simulink model "Main"  (Simulink 6.6)
settings: Solver=FixedStepDiscrete  StartTime=0.0  StopTime=Inf  FixedStep=0.001  RelTol=1e-3
undefined symbols (not defined in the file): ecan1_init, ecan1_receive_matlab, ecan1_transmit_matlab, u1, y1
libraries: simulink x83, dsPICdrivers x6
(part 1 of 2)
CloseFcn:
  | rtwprivate ssgencode ModelCloseRequest Main
settings Model: Creator=bwmairs  LastModifiedBy=bwmairs  ProdHWDeviceType=16-bit Generic
settings OptimizationCC: InlineParams=on  OptimizeModelRefInitCode=on  LifeSpan=1
settings HardwareCC: ProdBitPerInt=16  ProdEndianess=LittleEndian  ProdWordSize=16  ProdHWDeviceType=16-bit Generic  TargetHWDeviceType=32-bit Generic
settings RTWCC: SystemTargetFile=dspic.tlc  TemplateMakefile=dspic_pic30_gcc.tmf  PostCodeGenCommand=dsPIC_Compile()  Description=Embedded Target for Microchip dsPIC (real-time)  ProcessScript=dspic_make_rtw_hook
settings RTWCC: CustomSource=|
  | ../../circBuffer.c
  | ../../ecanFunctions.c
settings CodeAppCC: IgnoreCustomStorageClasses=off
settings STFCustomTargetCC: TargetFcnLib=ansi_tfl_tmw.mat  GenFloatMathFcnCalls=ANSI_C  ModelReferenceCompliant=off  IncludeMdlTerminateFcn=off  CombineOutputUpdateFcns=on  SuppressErrorStatus=on  ERTCustomFileBanners=on  SupportContinuousTime=off  SupportNonInlinedSFcns=off  SystemTargetFile=dspic.tlc
settings ERTTargetCC: TargetFcnLib=ansi_tfl_tmw.mat  GenFloatMathFcnCalls=ANSI_C  ModelReferenceCompliant=off  IncludeMdlTerminateFcn=off  SuppressErrorStatus=on  ModelStepFunctionPrototypeControlCompliant=off  ExtModeMexFile=noextcomm  InlinedParameterPlacement=NonHierarchical  ERTSrcFileBannerTemplate=dsPIC_code_template.cgt  ERTHdrFileBannerTemplate=dsPIC_code_template.cgt  ERTDataSrcFileTemplate=dsPIC_code_template.cgt  ERTDataHdrFileTemplate=dsPIC_code_template.cgt  ERTCustomFileTemplate=dsPIC_main.tlc
settings CustomProperty: DataType=string  Value=C:\PROGRA~1\MATLAB\R2007a\rtw\bin\win32\gmake

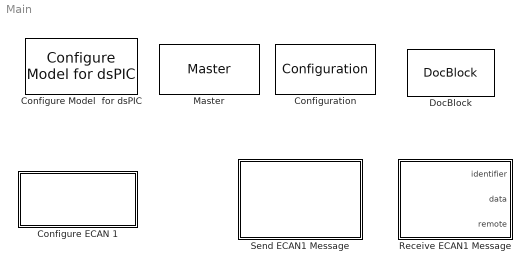
== system Main ==
  Configuration : dsPICdrivers/Configuration  SystemSampleTime=-1  double64=off
  Configure ECAN 1 : Subsystem  mask(Initialize ECAN 1){frame_setting=off, mode=Normal, dma_rx_chan=2, dma_tx_chan=0, baud=2500, cpu_freq=40000, ps1=8, pd=5, ps2=6, sjw=3, tq=20, triple_sample=on, dma_buf_size=4 buffers, rx_bufs=[0], tx_bufs=[1], buf_0_tx_pri=Highest, buf_0_rte=No, buf_1_tx_pri=Highest, buf_1_rte=No, buf_2_tx_pri=Lowest, buf_2_rte=No, buf_3_tx_pri=Lowest, buf_3_rte=No, buf_4_tx_pri=Lowest, buf_4_rte=No, buf_5_tx_pri=Lowest, buf_5_rte=No, buf_6_tx_pri=Lowest, buf_6_rte=No, buf_7_tx_pri=Lowest, buf_7_rte=No, mask_0=0, mask_0_rm=0, mask_1=0, mask_1_rm=0, mask_2=0, mask_2_rm=0, filters=[0 1 2], filter_0=hex2dec('400'), filter_0_mask=1, filter_0_exide=off, filter_0_buf=1, filter_1=hex2dec('401'), filter_1_mask=1, filter_1_exide=off, filter_1_buf=1, filter_2=hex2dec('402'), filter_2_mask=1, filter_2_exide=off, filter_2_buf=1, filter_3=0, filter_3_mask=0, filter_3_exide=off, filter_3_buf=0, filter_4=0, filter_4_mask=0, filter_4_exide=0, filter_4_buf=0, filter_5=0, filter_5_mask=0, filter_5_exide=off, filter_5_buf=0, filter_6=0, filter_6_mask=0, filter_6_exide=off, filter_6_buf=0, filter_7=0, filter_7_mask=0, filter_7_exide=off, filter_7_buf=0, filter_8=0, filter_8_mask=0, filter_8_exide=off, filter_8_buf=0, filter_9=0, filter_9_mask=0, filter_9_exide=off, filter_9_buf=0, filter_10=0, filter_10_mask=0, filter_10_exide=off, filter_10_buf=0, filter_11=0, filter_11_mask=0, filter_11_exide=off, filter_11_buf=0, filter_12=0, filter_12_mask=0, filter_12_exide=off, filter_12_buf=0, filter_13=0, filter_13_mask=0, filter_13_exide=off, filter_13_buf=0, filter_14=0, filter_14_mask=0, filter_14_exide=off, filter_14_buf=0, filter_15=0, filter_15_mask=0, filter_15_exide=off, filter_15_buf=0}
      mask prompts: frame_setting "Extended Frames (Standard if unchecked)"; dma_rx_chan "DMA Reception Channel"; dma_tx_chan "DMA Transmission Channel"; baud "Baud Rate (hundreds of bps)"; cpu_freq "CPU Frequency (in kHz)"; ps1 "Phase Segment 1"; pd "Propagation Delay"; ps2 "Phase Segment 2"; sjw "Sync Jump Width"; tq "Time Quanta"; triple_sample "Triple-sample"; dma_buf_size "DMA Buffer Size"; rx_bufs "Reception Buffers"; tx_bufs "Transmission Buffers"; buf_0_tx_pri "Buffer 0 Transmission Priority"; buf_0_rte "Buffer 0 Remote Transmit Enable"; buf_1_tx_pri "Buffer 1 Transmission Priority"; buf_1_rte "Buffer 1 Remote Transmit Enable"; buf_2_tx_pri "Buffer 2 Transmission Priority"; buf_2_rte "Buffer 2 Remote Transmit Enable"; buf_3_tx_pri "Buffer 3 Transmission Priority"; buf_3_rte "Buffer 3 Remote Transmit Enable"; buf_4_tx_pri "Buffer 4 Transmission Priority"; buf_4_rte "Buffer 4 Remote Transmit Enable"; buf_5_tx_pri "Buffer 5 Transmission Priority"; buf_5_rte "Buffer 5 Remote Transmit Enable"; buf_6_tx_pri "Buffer 6 Transmission Priority"; buf_6_rte "Buffer 6 Remote Transmit Enable"; buf_7_tx_pri "Buffer 7 Transmission Priority"; buf_7_rte "Buffer 7 Remote Transmit Enable"; mask_0 "Mask 0"; mask_0_rm "Mask 0 Receive Mode"; mask_1 "Mask 1"; mask_1_rm "Mask 1 Receive Mode"; mask_2 "Mask 2"; mask_2_rm "Mask 2 Receive Mode"; filter_0 "Filter 0"; filter_0_mask "Filter 0 Mask"; filter_0_exide "Filter 0 Extended Enable"; filter_0_buf "Filter 0 Buffer"; filter_1 "Filter 1"; filter_1_mask "Filter 1 Mask"; filter_1_exide "Filter 1 Extended Enable"; filter_1_buf "Filter 1 Buffer"; filter_2 "Filter 2"; filter_2_mask "Filter 2 Mask"; filter_2_exide "Filter 2 Extended Enable"; filter_2_buf "Filter 2 Buffer"; filter_3 "Filter 3"; filter_3_mask "Filter 3 Mask"; filter_3_exide "Filter 3 Extended Enable"; filter_3_buf "Filter 3 Buffer"; filter_4 "Filter 4"; filter_4_mask "Filter 4 Mask"; filter_4_exide "Filter 4 Extended Enable"; filter_4_buf "Filter 4 Buffer"; filter_5 "Filter 5"; filter_5_mask "Filter 5 Mask"; filter_5_exide "Filter 5 Extended Enable"; filter_5_buf "Filter 5 Buffer"; filter_6 "Filter 6"; filter_6_mask "Filter 6 Mask"; filter_6_exide "Filter 6 Extended Enable"; filter_6_buf "Filter 6 Buffer"; filter_7 "Filter 7"; filter_7_mask "Filter 7 Mask"; filter_7_exide "Filter 7 Extended Enable"; filter_7_buf "Filter 7 Buffer"; filter_8 "Filter 8"; filter_8_mask "Filter 8 Mask"; filter_8_exide "Filter 8 Extended Enable"; filter_8_buf "Filter 8 Buffer"; filter_9 "Filter 9"; filter_9_mask "Filter 9 Mask"; filter_9_exide "Filter 9 Extended Enable"; filter_9_buf "Filter 9 Buffer"; filter_10 "Filter 10"; filter_10_mask "Filter 10 Mask"; filter_10_exide "Filter 10 Extended Enable"; filter_10_buf "Filter 10 Buffer"; filter_11 "Filter 11"; filter_11_mask "Filter 11 Mask"; filter_11_exide "Filter 11 Extended Enable"; filter_11_buf "Filter 11 Buffer"; filter_12 "Filter 12"; filter_12_mask "Filter 12 Mask"; filter_12_exide "Filter 12 Extended Enable"; filter_12_buf "Filter 12 Buffer"; filter_13 "Filter 13"; filter_13_mask "Filter 13 Mask"; filter_13_exide "Filter 13 Extended Enable"; filter_13_buf "Filter 13 Buffer"; filter_14 "Filter 14"; filter_14_mask "Filter 14 Mask"; filter_14_exide "Filter 14 Extended Enable"; filter_14_buf "Filter 14 Buffer"; filter_15 "Filter 15"; filter_15_mask "Filter 15 Mask"; filter_15_exide "Filter 15 Extended Enable"; filter_15_buf "Filter 15 Buffer"
      mask help: Initializes the ECAN 1 module on the dsPIC33f. Allows for configuration of almost all ECAN options to produce a usable system.
      mask StyleString: checkbox,popup(Normal|Disabled|Loopback|Listen only|Configuration|UNDEFINED|UNDEFINED|Listen all),edit,edit,edit,edit,edit,edit,edit,popup(0|1|2|3),edit,checkbox,popup(4 buffers|6 buffers|8 buffers|12 buffers|16 buffers|24 buffers|32 buffers),edit,edit,popup(Lowest|Low|High|Highest),popup(No|Yes),popup(Lowest|Low|High|Highest),popup(No|Yes),popup(Lowest|Low|High|Highest),popup(No|Yes),popup(Lowest|Low|High|Highest),popup(No|Yes),popup(Lowest|Low|High|Highest),popup(No|Yes),popup(Lowest|Low|High|Highest),popup(No|Yes),popup(Lowest|Low|High|Highest),popup(No|Yes),popup(Lowest|Low|High|Highest),popup(No|Yes),edit,popup(0|1),edit,popup(0|1),edit,popup(0|1),edit,edit,popup(--|0|1|2),checkbox,popup(0|1|2|3|4|5|6|7|8|9|10|11|12|13|14|FIFO),edit,popup(0|1|2|--),checkbox,popup(0|1|2|3|4|5|6|7|8|9|10|11|12|13|14|FIFO),edit,popup(0|1|2|--),checkbox,popup(0|1|2|3|4|5|6|7|8|9|10|11|12|13|14|FIFO),edit,popup(0|1|2|--),checkbox,popup(0|1|2|3|4|5|6|7|8|9|10|11|12|13|14|FIFO),edit,popup(0|1|2|--),edit,popup(0|1|2|3|4|5|6|7|8|9|10|11|12|13|14|FIFO),edit,popup(0|1|2|--),checkbox,popup(0|1|2|3|4|5|6|7|8|9|10|11|12|13|14|FIFO),edit,popup(0|1|2|--),checkbox,popup(0|1|2|3|4|5|6|7|8|9|10|11|12|13|14|FIFO),edit,popup(0|1|2|--),checkbox,popup(0|1|2|3|4|5|6|7|8|9|10|11|12|13|14|FIFO),edit,popup(0|1|2|--),checkbox,popup(0|1|2|3|4|5|6|7|8|9|10|11|12|13|14|FIFO),edit,popup(0|1|2|--),checkbox,popup(0|1|2|3|4|5|6|7|8|9|10|11|12|13|14|FIFO),edit,popup(0|1|2|--),checkbox,popup(0|1|2|3|4|5|6|7|8|9|10|11|12|13|14|FIFO),edit,popup(0|1|2|--),checkbox,popup(0|1|2|3|4|5|6|7|8|9|10|11|12|13|14|FIFO),edit,popup(0|1|2|--),checkbox,popup(0|1|2|3|4|5|6|7|8|9|10|11|12|13|14|FIFO),edit,popup(0|1|2|--),checkbox,popup(0|1|2|3|4|5|6|7|8|9|10|11|12|13|14|FIFO),edit,popup(0|1|2|--),checkbox,popup(0|1|2|3|4|5|6|7|8|9|10|11|12|13|14|FIFO),edit,popup(0|1|2|--),checkbox,popup(0|1|2|3|4|5|6|7|8|9|10|11|12|13|14|FIFO)
      mask CallbackString:
      | ||||||tq = 1 + str2num(get_param(gcb, 'ps1')) + str2num(get_param(gcb, 'pd')) + str2num(get_param(gcb, 'ps2'));
      | set_param(gcb, 'tq', int2str(tq));|tq = 1 + str2num(get_param(gcb, 'ps1')) + str2num(get_param(gcb, 'pd')) + str2num(get_param(gcb, 'ps2'));
      | set_param(gcb, 'tq', int2str(tq));|tq = 1 + str2num(get_param(gcb, 'ps1')) + str2num(get_param(gcb, 'pd')) + str2num(get_param(gcb, 'ps2'));
      | set_param(gcb, 'tq', int2str(tq));||||||filters = eval(get_param(gcb,'tx_bufs'));
      | mVisibilities = get_param(gcb,'MaskVisibilities');
      | mNames = get_param(gcb,'MaskNames');
      | for i = 1:size(mNames);
      | 	n = mNames{i};
      |     if size(n,2) > 4 && strcmp(n(1:4), 'buf_') == 1
      |         filterNumber = sscanf(n, 'buf_%d');
      |         if isempty(find(filters == filterNumber, 1)) == 0
      |              mVisibilities{i} = 'on';
      |         else
      |              mVisibilities{i} = 'off';
      |         end
      |     end
      | end
      | set_param(gcb, 'MaskVisibilities', mVisibilities);|||||||||||||||||||||||filters = eval(get_param(gcb,'filters'));
      | mVisibilities = get_param(gcb,'MaskVisibilities');
      | mNames = get_param(gcb,'MaskNames');
      | for i = 1:size(mNames);
      | 	n = mNames{i};
      |     if size(n,2) > 7 && strcmp(n(1:7), 'filter_') == 1
      |         filterNumber = sscanf(n, 'filter_%d');
      |         if isempty(find(filters == filterNumber, 1)) == 0
      |              mVisibilities{i} = 'on';
      |         else
      |              mVisibilities{i} = 'off';
      |         end
      |     end
      | end
      | set_param(gcb, 'MaskVisibilities', mVisibilities);||||||||||||||||||||||||||||||||||||||||||||||||||||||||||||||||
      mask Display: text(0.5,0.5,'Configure ECAN1','horizontalAlignment','center','verticalAlignment','middle');
  Configure Model  for dsPIC : dsPICdrivers/Simulink Configuration/Configure Model  for dsPIC
  DocBlock : simulink/Model-Wide Utilities/DocBlock  SystemSampleTime=-1  DocumentType=Text
      content=|
      | This model recreates the Crosswire application note from Microchip.
      | The Debugging directory includes an MPLAB project that can compile and load
      | the MATLAB-generated code in order to facilitate debugging.
  Master : dsPICdrivers/Master  Tag=dsPIC_MASTER  Priority=1  TimeStepType=Timer1  picType=33fJ256GP710  fcy=40000000  Quartz_33f=8e6  PLLActive_33f=on  fcyDesired_33f=40000000  tmr1="[1  39999  0]"  tmr1Info="Time Step : 0.001  ;   Error : 0%  PR1=39999"  tmr2345="[0  0  0  0  0  0  0  0]"  tmr2345cfg=[-1 -1 -1 -1 -1 -1 -1 -1]  IOautoConf=on  typePort="[ 0  0  0  0  0  0  0  0  0  0  0  0  0  0  0  0  0  0  0  0  0  0  0  0  0  0  0  0  0  0  0  0  0  0  0  0  0  0  0  0  0  0  0  0  0  0  0  0  0  0  0  0  0  0  0  0  0  0  0  0  0  0  0  0  0  0  0  0  0  0  0  0  0  0  0  0  0  0  0  0  0  0  0  0  0  0  0  0  0  0  0  0  0  0  0  0  0  0  0  0  0  0  0  0  0  0  0  0  0  0  0  0 ]"  TRIS="[ 65535  65535  65535  65535  65535  65535  65535 ]"  ADPCFG=0  MasterBusyPort=None  MasterOverloadPort=None  FOSC=Quartz (XT - HS)  ClockSwitchMonitor=Both disabled  TempProtection_33f=TEMP_ON  FPBOR=<empty>  PWRT=disable  MCLR=<empty>  PowerSave=off  OverrideFcy=off  NewFcy=1e6  PR2345="[65535  65535  65535  65535  65535  65535  65535  65535]"
  Receive ECAN1 Message : Subsystem
  Send ECAN1 Message : Subsystem  mask(Send ECAN Message){buffer=1, identifier=hex2dec('401'), identifier_from_input=off, ide=off, remote=off, length=4, data=[hex2dec('11') hex2dec('12') hex2dec('13') hex2dec('14')], data_from_input=off, c_func_sample_time=1, trigger_on_input=off}
      mask prompts: identifier_from_input "Indentifier from input"; length "Data Length (bytes)"; data_from_input "Data from input"; c_func_sample_time "Sample time"; trigger_on_input "Trigger on input"
      mask help: This block allows for the transmission of a message over the ECAN module.
      mask CallbackString:
      | ||mEnables = get_param(gcb,'MaskEnables');
      | enabled = get_param(gcb, 'identifier_from_input');
      | if strcmp(enabled,'on');
      |     replace_block([gcb '/identifier'],'Constant','Inport','noprompt');
      |     mEnables{2} = 'off';
      |     set_param([gcb '/identifier'],'Port','1');
      | else
      |     replace_block([gcb '/identifier'],'Inport','Constant','noprompt');
      |     mEnables{2} = 'on';
      |     set_param([gcb '/identifier'],'Value','identifier');
      | end
      | set_param(gcb, 'MaskEnables', mEnables);
      | ||||data = eval(get_param(gcb, 'data'));
      | y = size(data,1);
      | x = size(data,2);
      | if y > 1 && x > 1
      |     error('Data must be a 1-dimensional vector')
      | else
      |     if or(x > 8, y > 8)
      |     error('Data cannot be larger than 8-bytes');
      |     end
      | end|mEnables = get_param(gcb,'MaskEnables');
      | enabled = get_param(gcb, 'data_from_input');
      | if strcmp(enabled,'on');
      |     mEnables{7} = 'off';
      |     replace_block([gcb '/data'],'Constant','Inport','noprompt');
      |     if strcmp(get_param([gcb '/identifier'],'BlockType'), 'Inport');
      |         set_param([gcb '/data'],'Port','2');
      |     else
      |         set_param([gcb '/data'],'Port','1');
      |     end
      | else
      |     mEnables{7} = 'on';
      |     replace_block([gcb '/data'],'Inport','Constant','noprompt');
      |     set_param([gcb '/data'],'Value','data');
      | end
      | set_param(gcb, 'MaskEnables', mEnables);||mEnables = get_param(gcb,'MaskEnables');
      | enabled = get_param(gcb, 'trigger_on_input');
      | if strcmp(enabled,'on');
      |     mEnables{9} = 'off';
      |     set_param([gcb '/C-function Call/ECAN1 Transmit'],'SampleTime','-1');
      |     replace_block([gcb '/trigger'],'Constant','Inport','noprompt');
      | else
      |     mEnables{9} = 'on';
      |     set_param([gcb '/C-function Call/ECAN1 Transmit'],'SampleTime','c_func_sample_time');
      |     replace_block([gcb '/trigger'],'Inport','Constant','noprompt');
      |     set_param([gcb '/trigger'],'Value','1');
      | end
      | set_param(gcb, 'MaskEnables', mEnables);
      mask Display: disp('ECAN1 TX');

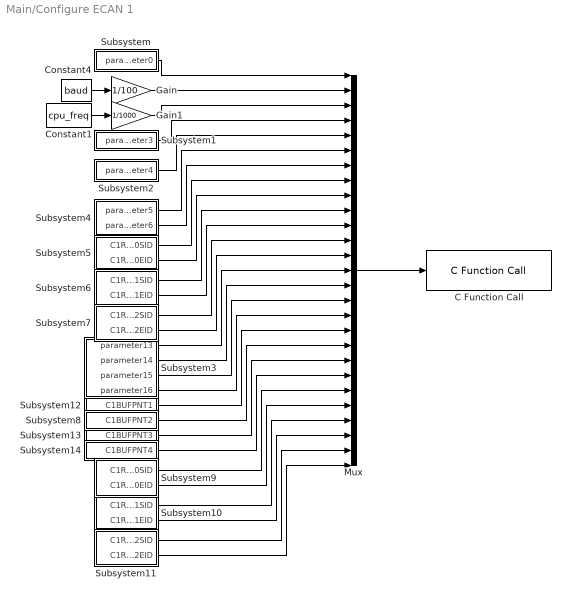
== system Main/Configure ECAN 1 ==
  C Function Call : dsPICdrivers/OTHERS/C Function Call  Tag=dsPIC_dsPIC_CFunctionCall  fctName='ecan1_init'  INPUT_SIZE=27  INPUT1=uint16  INPUT2=--  INPUT3=--  OUTPUT_SIZE=1  OUTPUT1=--  SampleTime=Inf  InputType=[ 4 ]  OutputType=[ ]  FctDeclaration=extern void ecan1_init(uint16_T* u1);  FctCall=ecan1_init(*%u1);  OrderingInOutPopup=None
  Constant1 : Constant  Value=cpu_freq  OutDataTypeMode=uint32
  Constant4 : Constant  Value=baud  OutDataTypeMode=uint32
  Gain : Gain  Gain=1/100  ParameterDataType=uint(16)  OutDataType=uint(16)
  Gain1 : Gain  Gain=1/1000  ParameterDataType=uint(16)
  Mux : Mux  Inputs=27
  Subsystem : Subsystem
  Subsystem1 : Subsystem
  Subsystem10 : Subsystem
  Subsystem11 : Subsystem
  Subsystem12 : Subsystem
  Subsystem13 : Subsystem
  Subsystem14 : Subsystem
  Subsystem2 : Subsystem
  Subsystem3 : Subsystem
  Subsystem4 : Subsystem
  Subsystem5 : Subsystem
  Subsystem6 : Subsystem
  Subsystem7 : Subsystem
  Subsystem8 : Subsystem
  Subsystem9 : Subsystem
  wires:
  Constant4/1 -> Gain/1
  Subsystem/1(parameter0) -> Mux/1
  Gain/1 -> Mux/2
  Subsystem1/1(parameter3) -> Mux/4
  Subsystem2/1(parameter4) -> Mux/5
  Subsystem4/2(parameter6) -> Mux/7
  Subsystem4/1(parameter5) -> Mux/6
  Subsystem5/1(C1RXM0SID) -> Mux/8
  Subsystem5/2(C1RXM0EID) -> Mux/9
  Subsystem6/1(C1RXM1SID) -> Mux/10
  Subsystem6/2(C1RXM1EID) -> Mux/11
  Subsystem7/1(C1RXM2SID) -> Mux/12
  Subsystem7/2(C1RXM2EID) -> Mux/13
  Subsystem3/1(parameter13) -> Mux/14
  Subsystem3/2(parameter14) -> Mux/15
  Subsystem3/3(parameter15) -> Mux/16
  Subsystem3/4(parameter16) -> Mux/17
  Subsystem12/1(C1BUFPNT1) -> Mux/18
  Subsystem8/1(C1BUFPNT2) -> Mux/19
  Subsystem13/1(C1BUFPNT3) -> Mux/20
  Subsystem14/1(C1BUFPNT4) -> Mux/21
  Subsystem9/1(C1RXF0SID) -> Mux/22
  Subsystem9/2(C1RXF0EID) -> Mux/23
  Subsystem10/1(C1RXF1SID) -> Mux/24
  Subsystem10/2(C1RXF1EID) -> Mux/25
  Subsystem11/1(C1RXF2SID) -> Mux/26
  Subsystem11/2(C1RXF2EID) -> Mux/27
  Constant1/1 -> Gain1/1
  Gain1/1 -> Mux/3
  Mux/1 -> C Function Call/1

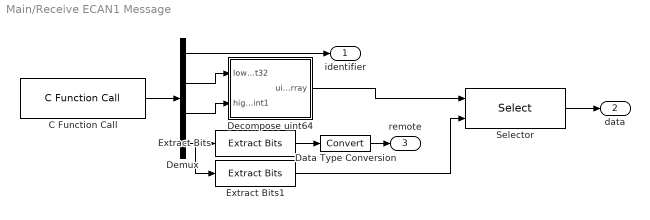
== system Main/Receive ECAN1 Message ==
  C Function Call : dsPICdrivers/OTHERS/C Function Call  Tag=dsPIC_dsPIC_CFunctionCall  fctName='ecan1_receive_matlab'  INPUT_SIZE=1  INPUT1=--  INPUT2=--  INPUT3=--  OUTPUT_SIZE=4  OUTPUT1=uint32  SampleTime=-1  InputType=[ ]  OutputType=[ 6 ]  FctDeclaration=extern void ecan1_receive_matlab(uint32_T* y1);  FctCall=ecan1_receive_matlab(*%y1);  OrderingInOutPopup=None
  Data Type Conversion : DataTypeConversion  OutDataTypeMode=boolean
  Decompose uint64 : Subsystem
  Demux : Demux
  Extract Bits : simulink/Logic and Bit Operations/Extract Bits  SystemSampleTime=-1  bitsToExtract=Lower half  numBits=8  bitIdxRange=[0 7]  outScalingMode=Treat bit field as an integer
  Extract Bits1 : simulink/Logic and Bit Operations/Extract Bits  SystemSampleTime=-1  bitsToExtract=Upper half  numBits=8  bitIdxRange=[0 7]  outScalingMode=Treat bit field as an integer
  Selector : Selector  IndexMode=Zero-based  IndexOptions=Index vector (port)  Indices=[1 3]  OutputSizes=1  InputPortWidth=8
  identifier : Outport
  data : Outport  Port=2
  remote : Outport  Port=3
  wires:
  C Function Call/1 -> Demux/1
  Demux/1 -> identifier/1
  Demux/3 -> Decompose uint64/2(high-order uint1)
  Demux/4 -> Extract Bits/1, Extract Bits1/1
  Data Type Conversion/1 -> remote/1
  Demux/2 -> Decompose uint64/1(low-order uint32)
  Extract Bits/1 -> Data Type Conversion/1
  Selector/1 -> data/1
  Decompose uint64/1(uint8 array) -> Selector/1
  Extract Bits1/1 -> Selector/2

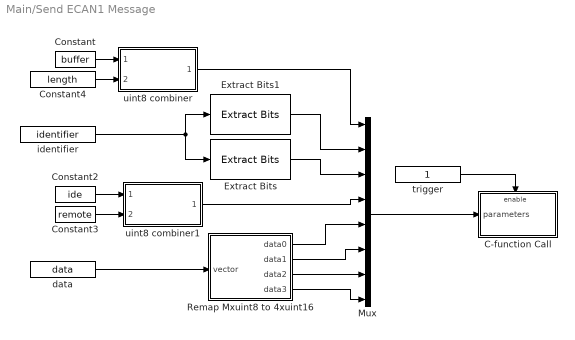
== system Main/Send ECAN1 Message ==
  C-function Call : Subsystem
  Constant : Constant  Value=buffer  OutDataTypeMode=uint16
  Constant2 : Constant  Value=ide  OutDataTypeMode=uint16
  Constant3 : Constant  Value=remote  OutDataTypeMode=uint16
  Constant4 : Constant  Value=length  OutDataTypeMode=uint16
  Extract Bits : simulink/Logic and Bit Operations/Extract Bits  SystemSampleTime=-1  bitsToExtract=Upper half  numBits=8  bitIdxRange=[0 7]  outScalingMode=Treat bit field as an integer
  Extract Bits1 : simulink/Logic and Bit Operations/Extract Bits  SystemSampleTime=-1  bitsToExtract=Lower half  numBits=8  bitIdxRange=[0 7]  outScalingMode=Preserve fixed-point scaling
  Mux : Mux  Inputs=8
  Remap Mxuint8 to 4xuint16 : Subsystem
  data : Constant  Value=data  OutDataTypeMode=uint8
  identifier : Constant  Value=identifier  OutDataTypeMode=uint32
  trigger : Constant  OutDataTypeMode=boolean
  uint8 combiner : Subsystem
  uint8 combiner1 : Subsystem
  wires:
  trigger/1 -> C-function Call/Enable
  Mux/1 -> C-function Call/1(parameters)
  uint8 combiner/1(combined) -> Mux/1
  Constant/1 -> uint8 combiner/1(high-order)
  Constant4/1 -> uint8 combiner/2(low-order)
  Extract Bits/1 -> Mux/3
  Extract Bits1/1 -> Mux/2
  identifier/1 -> Extract Bits1/1, Extract Bits/1
  uint8 combiner1/1(combined) -> Mux/4
  Constant3/1 -> uint8 combiner1/2(low-order)
  Constant2/1 -> uint8 combiner1/1(high-order)
  Remap Mxuint8 to 4xuint16/1(data0) -> Mux/5
  Remap Mxuint8 to 4xuint16/2(data1) -> Mux/6
  Remap Mxuint8 to 4xuint16/3(data2) -> Mux/7
  Remap Mxuint8 to 4xuint16/4(data3) -> Mux/8
  data/1 -> Remap Mxuint8 to 4xuint16/1(vector)

== system Main/Configure ECAN 1/Subsystem ==
  Constant : Constant  Value=frame_setting  OutDataTypeMode=uint16
  Constant1 : Constant  Value=mode  OutDataTypeMode=uint16
  Constant2 : Constant  Value=dma_rx_chan  OutDataTypeMode=uint16
  Constant3 : Constant  Value=dma_tx_chan  OutDataTypeMode=uint16
  Logical Operator : Logic  Operator=OR  Inputs=4  OutDataTypeMode=Specify via dialog  LogicDataType=uint(16)
  Shift Arithmetic1 : simulink/Logic and Bit Operations/Shift Arithmetic  SystemSampleTime=-1  nBitShiftRight=-2  nBinPtShiftRight=0
  Shift Arithmetic2 : simulink/Logic and Bit Operations/Shift Arithmetic  SystemSampleTime=-1  nBitShiftRight=-5  nBinPtShiftRight=0
  Shift Arithmetic3 : simulink/Logic and Bit Operations/Shift Arithmetic  SystemSampleTime=-1  nBitShiftRight=-8  nBinPtShiftRight=0
  parameter0 : Outport
  wires:
  Shift Arithmetic1/1 -> Logical Operator/2
  Shift Arithmetic2/1 -> Logical Operator/3
  Shift Arithmetic3/1 -> Logical Operator/4
  Logical Operator/1 -> parameter0/1
  Constant3/1 -> Shift Arithmetic3/1
  Constant2/1 -> Shift Arithmetic2/1
  Constant1/1 -> Shift Arithmetic1/1
  Constant/1 -> Logical Operator/1

== system Main/Configure ECAN 1/Subsystem1 ==
  Constant1 : Constant  Value=sjw  OutDataTypeMode=uint16
  Constant2 : Constant  Value=triple_sample  OutDataTypeMode=uint16
  Constant5 : Constant  Value=ps1  OutDataTypeMode=uint16
  Constant6 : Constant  Value=pd  OutDataTypeMode=uint16
  Constant7 : Constant  Value=ps2  OutDataTypeMode=uint16
  Logical Operator : Logic  Operator=OR  Inputs=5  OutDataTypeMode=Specify via dialog  LogicDataType=uint(16)
  Shift Arithmetic1 : simulink/Logic and Bit Operations/Shift Arithmetic  SystemSampleTime=-1  nBitShiftRight=-3  nBinPtShiftRight=0
  Shift Arithmetic2 : simulink/Logic and Bit Operations/Shift Arithmetic  SystemSampleTime=-1  nBitShiftRight=-6  nBinPtShiftRight=0
  Shift Arithmetic3 : simulink/Logic and Bit Operations/Shift Arithmetic  SystemSampleTime=-1  nBitShiftRight=-9  nBinPtShiftRight=0
  parameter3 : Outport
  wires:
  Shift Arithmetic1/1 -> Logical Operator/2
  Shift Arithmetic2/1 -> Logical Operator/3
  Logical Operator/1 -> parameter3/1
  Constant5/1 -> Logical Operator/1
  Constant6/1 -> Shift Arithmetic1/1
  Constant7/1 -> Shift Arithmetic2/1
  Shift Arithmetic3/1 -> Logical Operator/4
  Constant1/1 -> Shift Arithmetic3/1
  Constant2/1 -> Logical Operator/5

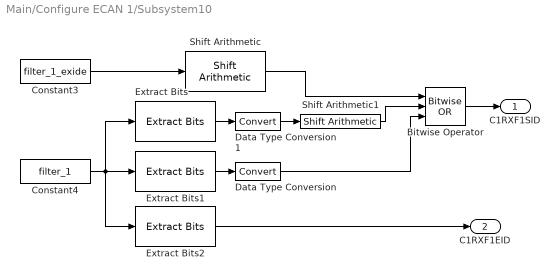
== system Main/Configure ECAN 1/Subsystem10 ==
  Bitwise Operator : simulink/Logic and Bit Operations/Bitwise Operator  logicop=OR  UseBitMask=off  NumInputPorts=3  BitMask=bin2dec('11011001')  BitMaskRealWorld=Stored Integer
  Constant3 : Constant  Value=filter_1_exide  OutDataTypeMode=uint16
  Constant4 : Constant  Value=filter_1  OutDataTypeMode=uint32
  Data Type Conversion : DataTypeConversion  OutDataTypeMode=uint16
  Data Type Conversion1 : DataTypeConversion  OutDataTypeMode=uint16
  Extract Bits : simulink/Logic and Bit Operations/Extract Bits  SystemSampleTime=-1  bitsToExtract=Range of bits  numBits=8  bitIdxRange=[0 11]  outScalingMode=Treat bit field as an integer
  Extract Bits1 : simulink/Logic and Bit Operations/Extract Bits  SystemSampleTime=-1  bitsToExtract=Range of bits  numBits=8  bitIdxRange=[0 1]  outScalingMode=Treat bit field as an integer
  Extract Bits2 : simulink/Logic and Bit Operations/Extract Bits  SystemSampleTime=-1  bitsToExtract=Range of bits  numBits=8  bitIdxRange=[11 26]  outScalingMode=Treat bit field as an integer
  Shift Arithmetic : simulink/Logic and Bit Operations/Shift Arithmetic  SystemSampleTime=-1  nBitShiftRight=-3  nBinPtShiftRight=0
  Shift Arithmetic1 : simulink/Logic and Bit Operations/Shift Arithmetic  SystemSampleTime=-1  nBitShiftRight=-5  nBinPtShiftRight=0
  C1RXF1SID : Outport
  C1RXF1EID : Outport  Port=2
  wires:
  Data Type Conversion/1 -> Bitwise Operator/3
  Extract Bits2/1 -> C1RXF1EID/1
  Extract Bits1/1 -> Data Type Conversion/1
  Constant4/1 -> Extract Bits2/1, Extract Bits1/1, Extract Bits/1
  Bitwise Operator/1 -> C1RXF1SID/1
  Shift Arithmetic1/1 -> Bitwise Operator/2
  Extract Bits/1 -> Data Type Conversion1/1
  Shift Arithmetic/1 -> Bitwise Operator/1
  Constant3/1 -> Shift Arithmetic/1
  Data Type Conversion1/1 -> Shift Arithmetic1/1

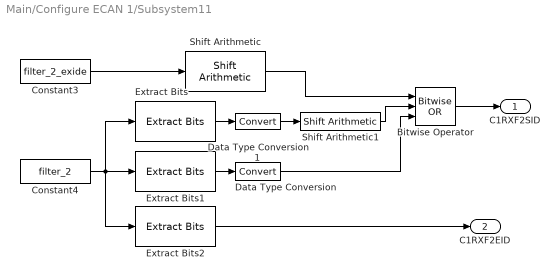
== system Main/Configure ECAN 1/Subsystem11 ==
  Bitwise Operator : simulink/Logic and Bit Operations/Bitwise Operator  logicop=OR  UseBitMask=off  NumInputPorts=3  BitMask=bin2dec('11011001')  BitMaskRealWorld=Stored Integer
  Constant3 : Constant  Value=filter_2_exide  OutDataTypeMode=uint16
  Constant4 : Constant  Value=filter_2  OutDataTypeMode=uint32
  Data Type Conversion : DataTypeConversion  OutDataTypeMode=uint16
  Data Type Conversion1 : DataTypeConversion  OutDataTypeMode=uint16
  Extract Bits : simulink/Logic and Bit Operations/Extract Bits  SystemSampleTime=-1  bitsToExtract=Range of bits  numBits=8  bitIdxRange=[0 11]  outScalingMode=Treat bit field as an integer
  Extract Bits1 : simulink/Logic and Bit Operations/Extract Bits  SystemSampleTime=-1  bitsToExtract=Range of bits  numBits=8  bitIdxRange=[0 1]  outScalingMode=Treat bit field as an integer
  Extract Bits2 : simulink/Logic and Bit Operations/Extract Bits  SystemSampleTime=-1  bitsToExtract=Range of bits  numBits=8  bitIdxRange=[11 26]  outScalingMode=Treat bit field as an integer
  Shift Arithmetic : simulink/Logic and Bit Operations/Shift Arithmetic  SystemSampleTime=-1  nBitShiftRight=-3  nBinPtShiftRight=0
  Shift Arithmetic1 : simulink/Logic and Bit Operations/Shift Arithmetic  SystemSampleTime=-1  nBitShiftRight=-5  nBinPtShiftRight=0
  C1RXF2SID : Outport
  C1RXF2EID : Outport  Port=2
  wires:
  Constant3/1 -> Shift Arithmetic/1
  Shift Arithmetic/1 -> Bitwise Operator/1
  Extract Bits/1 -> Data Type Conversion1/1
  Shift Arithmetic1/1 -> Bitwise Operator/2
  Bitwise Operator/1 -> C1RXF2SID/1
  Constant4/1 -> Extract Bits/1, Extract Bits1/1, Extract Bits2/1
  Extract Bits1/1 -> Data Type Conversion/1
  Extract Bits2/1 -> C1RXF2EID/1
  Data Type Conversion/1 -> Bitwise Operator/3
  Data Type Conversion1/1 -> Shift Arithmetic1/1

== system Main/Configure ECAN 1/Subsystem12 ==
  Bitwise Operator : simulink/Logic and Bit Operations/Bitwise Operator  logicop=OR  UseBitMask=off  NumInputPorts=4  BitMask=bin2dec('11011001')  BitMaskRealWorld=Stored Integer
  Constant : Constant  Value=filter_0_buf  OutDataTypeMode=uint16
  Constant2 : Constant  Value=filter_2_buf  OutDataTypeMode=uint16
  Constant3 : Constant  Value=filter_1_buf  OutDataTypeMode=uint16
  Constant5 : Constant  Value=filter_3_buf  OutDataTypeMode=uint16
  Shift Arithmetic : simulink/Logic and Bit Operations/Shift Arithmetic  SystemSampleTime=-1  nBitShiftRight=-4  nBinPtShiftRight=0
  Shift Arithmetic1 : simulink/Logic and Bit Operations/Shift Arithmetic  SystemSampleTime=-1  nBitShiftRight=-8  nBinPtShiftRight=0
  Shift Arithmetic2 : simulink/Logic and Bit Operations/Shift Arithmetic  SystemSampleTime=-1  nBitShiftRight=-12  nBinPtShiftRight=0
  C1BUFPNT1 : Outport
  wires:
  Constant3/1 -> Shift Arithmetic/1
  Constant2/1 -> Shift Arithmetic1/1
  Shift Arithmetic1/1 -> Bitwise Operator/3
  Constant5/1 -> Shift Arithmetic2/1
  Shift Arithmetic2/1 -> Bitwise Operator/4
  Constant/1 -> Bitwise Operator/1
  Bitwise Operator/1 -> C1BUFPNT1/1
  Shift Arithmetic/1 -> Bitwise Operator/2

== system Main/Configure ECAN 1/Subsystem13 ==
  Bitwise Operator : simulink/Logic and Bit Operations/Bitwise Operator  logicop=OR  UseBitMask=off  NumInputPorts=4  BitMask=bin2dec('11011001')  BitMaskRealWorld=Stored Integer
  Constant : Constant  Value=filter_8_buf  OutDataTypeMode=uint16
  Constant2 : Constant  Value=filter_10_buf  OutDataTypeMode=uint16
  Constant3 : Constant  Value=filter_9_buf  OutDataTypeMode=uint16
  Constant5 : Constant  Value=filter_11_buf  OutDataTypeMode=uint16
  Shift Arithmetic : simulink/Logic and Bit Operations/Shift Arithmetic  SystemSampleTime=-1  nBitShiftRight=-4  nBinPtShiftRight=0
  Shift Arithmetic1 : simulink/Logic and Bit Operations/Shift Arithmetic  SystemSampleTime=-1  nBitShiftRight=-8  nBinPtShiftRight=0
  Shift Arithmetic2 : simulink/Logic and Bit Operations/Shift Arithmetic  SystemSampleTime=-1  nBitShiftRight=-12  nBinPtShiftRight=0
  C1BUFPNT3 : Outport
  wires:
  Constant3/1 -> Shift Arithmetic/1
  Constant2/1 -> Shift Arithmetic1/1
  Shift Arithmetic1/1 -> Bitwise Operator/3
  Constant5/1 -> Shift Arithmetic2/1
  Shift Arithmetic2/1 -> Bitwise Operator/4
  Constant/1 -> Bitwise Operator/1
  Bitwise Operator/1 -> C1BUFPNT3/1
  Shift Arithmetic/1 -> Bitwise Operator/2

== system Main/Configure ECAN 1/Subsystem14 ==
  Bitwise Operator : simulink/Logic and Bit Operations/Bitwise Operator  logicop=OR  UseBitMask=off  NumInputPorts=4  BitMask=bin2dec('11011001')  BitMaskRealWorld=Stored Integer
  Constant : Constant  Value=filter_12_buf  OutDataTypeMode=uint16
  Constant2 : Constant  Value=filter_14_buf  OutDataTypeMode=uint16
  Constant3 : Constant  Value=filter_13_buf  OutDataTypeMode=uint16
  Constant5 : Constant  Value=filter_15_buf  OutDataTypeMode=uint16
  Shift Arithmetic : simulink/Logic and Bit Operations/Shift Arithmetic  SystemSampleTime=-1  nBitShiftRight=-4  nBinPtShiftRight=0
  Shift Arithmetic1 : simulink/Logic and Bit Operations/Shift Arithmetic  SystemSampleTime=-1  nBitShiftRight=-8  nBinPtShiftRight=0
  Shift Arithmetic2 : simulink/Logic and Bit Operations/Shift Arithmetic  SystemSampleTime=-1  nBitShiftRight=-12  nBinPtShiftRight=0
  C1BUFPNT4 : Outport
  wires:
  Shift Arithmetic/1 -> Bitwise Operator/2
  Bitwise Operator/1 -> C1BUFPNT4/1
  Constant/1 -> Bitwise Operator/1
  Shift Arithmetic2/1 -> Bitwise Operator/4
  Constant5/1 -> Shift Arithmetic2/1
  Shift Arithmetic1/1 -> Bitwise Operator/3
  Constant2/1 -> Shift Arithmetic1/1
  Constant3/1 -> Shift Arithmetic/1

== system Main/Configure ECAN 1/Subsystem2 ==
  Constant1 : Constant  Value=filters  OutDataTypeMode=uint16
  Embedded MATLAB Function : Stateflow chart
  parameter4 : Outport
  wires:
  Constant1/1 -> Embedded MATLAB Function/1(u)
  Embedded MATLAB Function/1(y) -> parameter4/1

== system Main/Configure ECAN 1/Subsystem3 ==
  Constant : Constant  Value=tx_bufs  OutDataTypeMode=uint16
  Constant1 : Constant  Value=[buf_0_tx_pri;buf_1_tx_pri;buf_2_tx_pri;buf_3_tx_pri;buf_4_tx_pri;buf_5_tx_pri;buf_6_tx_pri;buf_7_tx_pri]  VectorParams1D=off  OutDataTypeMode=uint16
  Constant2 : Constant  Value=[buf_0_rte;buf_1_rte;buf_2_rte;buf_3_rte;buf_4_rte;buf_5_rte;buf_6_rte;buf_7_rte]  OutDataTypeMode=uint16
  Embedded MATLAB Function : Stateflow chart
  parameter13 : Outport
  parameter14 : Outport  Port=2
  parameter15 : Outport  Port=3
  parameter16 : Outport  Port=4
  wires:
  Embedded MATLAB Function/2(CiTR23CON) -> parameter14/1
  Embedded MATLAB Function/1(CiTR01CON) -> parameter13/1
  Embedded MATLAB Function/3(CiTR45CON) -> parameter15/1
  Embedded MATLAB Function/4(CiTR67CON) -> parameter16/1
  Constant/1 -> Embedded MATLAB Function/1(bufs)
  Constant1/1 -> Embedded MATLAB Function/2(buf_priorities)
  Constant2/1 -> Embedded MATLAB Function/3(buf_rtes)

== system Main/Configure ECAN 1/Subsystem4 ==
  Constant1 : Constant  Value=[filter_0_mask filter_1_mask filter_2_mask filter_3_mask filter_4_mask filter_5_mask filter_6_mask filter_7_mask filter_8_mask filter_9_mask filter_10_mask filter_11_mask filter_12_mask filter_13_mask filter_14_mask filter_15_mask]  OutDataTypeMode=uint16
  Constant2 : Constant  Value=filters  OutDataTypeMode=uint16
  Embedded MATLAB Function : Stateflow chart
  parameter5 : Outport
  parameter6 : Outport  Port=2
  wires:
  Embedded MATLAB Function/2(sel2) -> parameter6/1
  Embedded MATLAB Function/1(sel1) -> parameter5/1
  Constant1/1 -> Embedded MATLAB Function/2(filter_masks)
  Constant2/1 -> Embedded MATLAB Function/1(filters)

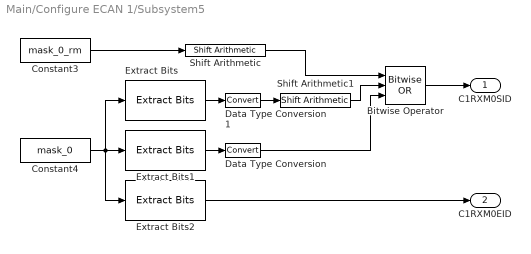
== system Main/Configure ECAN 1/Subsystem5 ==
  Bitwise Operator : simulink/Logic and Bit Operations/Bitwise Operator  logicop=OR  UseBitMask=off  NumInputPorts=3  BitMask=bin2dec('11011001')  BitMaskRealWorld=Stored Integer
  Constant3 : Constant  Value=mask_0_rm  OutDataTypeMode=uint16
  Constant4 : Constant  Value=mask_0  OutDataTypeMode=uint32
  Data Type Conversion : DataTypeConversion  OutDataTypeMode=uint16
  Data Type Conversion1 : DataTypeConversion  OutDataTypeMode=uint16
  Extract Bits : simulink/Logic and Bit Operations/Extract Bits  SystemSampleTime=-1  bitsToExtract=Range of bits  numBits=8  bitIdxRange=[0 11]  outScalingMode=Treat bit field as an integer
  Extract Bits1 : simulink/Logic and Bit Operations/Extract Bits  SystemSampleTime=-1  bitsToExtract=Range of bits  numBits=8  bitIdxRange=[0 1]  outScalingMode=Treat bit field as an integer
  Extract Bits2 : simulink/Logic and Bit Operations/Extract Bits  SystemSampleTime=-1  bitsToExtract=Range of bits  numBits=8  bitIdxRange=[11 26]  outScalingMode=Treat bit field as an integer
  Shift Arithmetic : simulink/Logic and Bit Operations/Shift Arithmetic  SystemSampleTime=-1  nBitShiftRight=-3  nBinPtShiftRight=0
  Shift Arithmetic1 : simulink/Logic and Bit Operations/Shift Arithmetic  SystemSampleTime=-1  nBitShiftRight=-5  nBinPtShiftRight=0
  C1RXM0SID : Outport
  C1RXM0EID : Outport  Port=2
  wires:
  Constant3/1 -> Shift Arithmetic/1
  Shift Arithmetic/1 -> Bitwise Operator/1
  Extract Bits/1 -> Data Type Conversion1/1
  Shift Arithmetic1/1 -> Bitwise Operator/2
  Bitwise Operator/1 -> C1RXM0SID/1
  Constant4/1 -> Extract Bits/1, Extract Bits1/1, Extract Bits2/1
  Extract Bits1/1 -> Data Type Conversion/1
  Extract Bits2/1 -> C1RXM0EID/1
  Data Type Conversion/1 -> Bitwise Operator/3
  Data Type Conversion1/1 -> Shift Arithmetic1/1

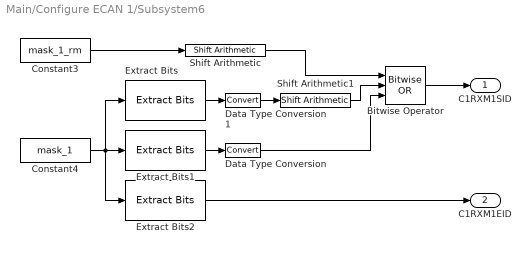
== system Main/Configure ECAN 1/Subsystem6 ==
  Bitwise Operator : simulink/Logic and Bit Operations/Bitwise Operator  logicop=OR  UseBitMask=off  NumInputPorts=3  BitMask=bin2dec('11011001')  BitMaskRealWorld=Stored Integer
  Constant3 : Constant  Value=mask_1_rm  OutDataTypeMode=uint16
  Constant4 : Constant  Value=mask_1  OutDataTypeMode=uint32
  Data Type Conversion : DataTypeConversion  OutDataTypeMode=uint16
  Data Type Conversion1 : DataTypeConversion  OutDataTypeMode=uint16
  Extract Bits : simulink/Logic and Bit Operations/Extract Bits  SystemSampleTime=-1  bitsToExtract=Range of bits  numBits=8  bitIdxRange=[0 11]  outScalingMode=Treat bit field as an integer
  Extract Bits1 : simulink/Logic and Bit Operations/Extract Bits  SystemSampleTime=-1  bitsToExtract=Range of bits  numBits=8  bitIdxRange=[0 1]  outScalingMode=Treat bit field as an integer
  Extract Bits2 : simulink/Logic and Bit Operations/Extract Bits  SystemSampleTime=-1  bitsToExtract=Range of bits  numBits=8  bitIdxRange=[11 26]  outScalingMode=Treat bit field as an integer
  Shift Arithmetic : simulink/Logic and Bit Operations/Shift Arithmetic  SystemSampleTime=-1  nBitShiftRight=-3  nBinPtShiftRight=0
  Shift Arithmetic1 : simulink/Logic and Bit Operations/Shift Arithmetic  SystemSampleTime=-1  nBitShiftRight=-5  nBinPtShiftRight=0
  C1RXM1SID : Outport
  C1RXM1EID : Outport  Port=2
  wires:
  Constant3/1 -> Shift Arithmetic/1
  Shift Arithmetic/1 -> Bitwise Operator/1
  Extract Bits/1 -> Data Type Conversion1/1
  Shift Arithmetic1/1 -> Bitwise Operator/2
  Bitwise Operator/1 -> C1RXM1SID/1
  Constant4/1 -> Extract Bits/1, Extract Bits1/1, Extract Bits2/1
  Extract Bits1/1 -> Data Type Conversion/1
  Extract Bits2/1 -> C1RXM1EID/1
  Data Type Conversion/1 -> Bitwise Operator/3
  Data Type Conversion1/1 -> Shift Arithmetic1/1

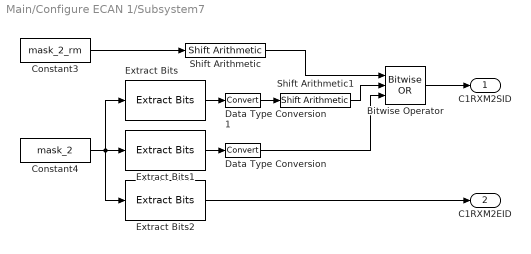
== system Main/Configure ECAN 1/Subsystem7 ==
  Bitwise Operator : simulink/Logic and Bit Operations/Bitwise Operator  logicop=OR  UseBitMask=off  NumInputPorts=3  BitMask=bin2dec('11011001')  BitMaskRealWorld=Stored Integer
  Constant3 : Constant  Value=mask_2_rm  OutDataTypeMode=uint16
  Constant4 : Constant  Value=mask_2  OutDataTypeMode=uint32
  Data Type Conversion : DataTypeConversion  OutDataTypeMode=uint16
  Data Type Conversion1 : DataTypeConversion  OutDataTypeMode=uint16
  Extract Bits : simulink/Logic and Bit Operations/Extract Bits  SystemSampleTime=-1  bitsToExtract=Range of bits  numBits=8  bitIdxRange=[0 11]  outScalingMode=Treat bit field as an integer
  Extract Bits1 : simulink/Logic and Bit Operations/Extract Bits  SystemSampleTime=-1  bitsToExtract=Range of bits  numBits=8  bitIdxRange=[0 1]  outScalingMode=Treat bit field as an integer
  Extract Bits2 : simulink/Logic and Bit Operations/Extract Bits  SystemSampleTime=-1  bitsToExtract=Range of bits  numBits=8  bitIdxRange=[11 26]  outScalingMode=Treat bit field as an integer
  Shift Arithmetic : simulink/Logic and Bit Operations/Shift Arithmetic  SystemSampleTime=-1  nBitShiftRight=-3  nBinPtShiftRight=0
  Shift Arithmetic1 : simulink/Logic and Bit Operations/Shift Arithmetic  SystemSampleTime=-1  nBitShiftRight=-5  nBinPtShiftRight=0
  C1RXM2SID : Outport
  C1RXM2EID : Outport  Port=2
  wires:
  Constant3/1 -> Shift Arithmetic/1
  Shift Arithmetic/1 -> Bitwise Operator/1
  Extract Bits/1 -> Data Type Conversion1/1
  Shift Arithmetic1/1 -> Bitwise Operator/2
  Bitwise Operator/1 -> C1RXM2SID/1
  Constant4/1 -> Extract Bits/1, Extract Bits1/1, Extract Bits2/1
  Extract Bits1/1 -> Data Type Conversion/1
  Extract Bits2/1 -> C1RXM2EID/1
  Data Type Conversion/1 -> Bitwise Operator/3
  Data Type Conversion1/1 -> Shift Arithmetic1/1

== system Main/Configure ECAN 1/Subsystem8 ==
  Bitwise Operator : simulink/Logic and Bit Operations/Bitwise Operator  logicop=OR  UseBitMask=off  NumInputPorts=4  BitMask=bin2dec('11011001')  BitMaskRealWorld=Stored Integer
  Constant : Constant  Value=filter_4_buf  OutDataTypeMode=uint16
  Constant2 : Constant  Value=filter_6_buf  OutDataTypeMode=uint16
  Constant3 : Constant  Value=filter_5_buf  OutDataTypeMode=uint16
  Constant5 : Constant  Value=filter_7_buf  OutDataTypeMode=uint16
  Shift Arithmetic : simulink/Logic and Bit Operations/Shift Arithmetic  SystemSampleTime=-1  nBitShiftRight=-4  nBinPtShiftRight=0
  Shift Arithmetic1 : simulink/Logic and Bit Operations/Shift Arithmetic  SystemSampleTime=-1  nBitShiftRight=-8  nBinPtShiftRight=0
  Shift Arithmetic2 : simulink/Logic and Bit Operations/Shift Arithmetic  SystemSampleTime=-1  nBitShiftRight=-12  nBinPtShiftRight=0
  C1BUFPNT2 : Outport
  wires:
  Shift Arithmetic/1 -> Bitwise Operator/2
  Bitwise Operator/1 -> C1BUFPNT2/1
  Constant/1 -> Bitwise Operator/1
  Shift Arithmetic2/1 -> Bitwise Operator/4
  Constant5/1 -> Shift Arithmetic2/1
  Shift Arithmetic1/1 -> Bitwise Operator/3
  Constant2/1 -> Shift Arithmetic1/1
  Constant3/1 -> Shift Arithmetic/1

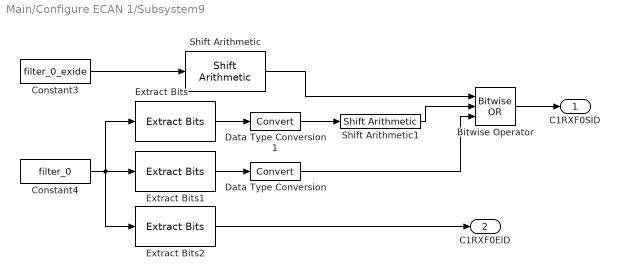
== system Main/Configure ECAN 1/Subsystem9 ==
  Bitwise Operator : simulink/Logic and Bit Operations/Bitwise Operator  logicop=OR  UseBitMask=off  NumInputPorts=3  BitMask=bin2dec('11011001')  BitMaskRealWorld=Stored Integer
  Constant3 : Constant  Value=filter_0_exide  OutDataTypeMode=uint16
  Constant4 : Constant  Value=filter_0  OutDataTypeMode=uint32
  Data Type Conversion : DataTypeConversion  OutDataTypeMode=uint16
  Data Type Conversion1 : DataTypeConversion  OutDataTypeMode=uint16
  Extract Bits : simulink/Logic and Bit Operations/Extract Bits  SystemSampleTime=-1  bitsToExtract=Range of bits  numBits=8  bitIdxRange=[0 11]  outScalingMode=Treat bit field as an integer
  Extract Bits1 : simulink/Logic and Bit Operations/Extract Bits  SystemSampleTime=-1  bitsToExtract=Range of bits  numBits=8  bitIdxRange=[0 1]  outScalingMode=Treat bit field as an integer
  Extract Bits2 : simulink/Logic and Bit Operations/Extract Bits  SystemSampleTime=-1  bitsToExtract=Range of bits  numBits=8  bitIdxRange=[11 26]  outScalingMode=Treat bit field as an integer
  Shift Arithmetic : simulink/Logic and Bit Operations/Shift Arithmetic  SystemSampleTime=-1  nBitShiftRight=-3  nBinPtShiftRight=0
  Shift Arithmetic1 : simulink/Logic and Bit Operations/Shift Arithmetic  SystemSampleTime=-1  nBitShiftRight=-5  nBinPtShiftRight=0
  C1RXF0SID : Outport
  C1RXF0EID : Outport  Port=2
  wires:
  Constant3/1 -> Shift Arithmetic/1
  Shift Arithmetic/1 -> Bitwise Operator/1
  Extract Bits/1 -> Data Type Conversion1/1
  Shift Arithmetic1/1 -> Bitwise Operator/2
  Bitwise Operator/1 -> C1RXF0SID/1
  Constant4/1 -> Extract Bits/1, Extract Bits1/1, Extract Bits2/1
  Extract Bits1/1 -> Data Type Conversion/1
  Extract Bits2/1 -> C1RXF0EID/1
  Data Type Conversion/1 -> Bitwise Operator/3
  Data Type Conversion1/1 -> Shift Arithmetic1/1

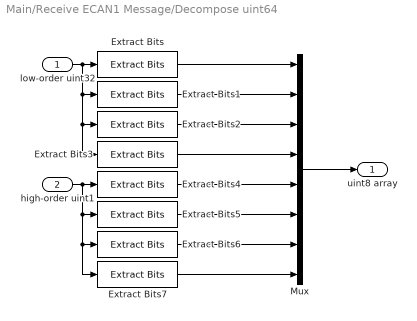
== system Main/Receive ECAN1 Message/Decompose uint64 ==
  low-order uint32 : Inport
  high-order uint1 : Inport  Port=2
  Extract Bits : simulink/Logic and Bit Operations/Extract Bits  SystemSampleTime=-1  bitsToExtract=Range of bits  numBits=8  bitIdxRange=[0 7]  outScalingMode=Treat bit field as an integer
  Extract Bits1 : simulink/Logic and Bit Operations/Extract Bits  SystemSampleTime=-1  bitsToExtract=Range of bits  numBits=8  bitIdxRange=[8 15]  outScalingMode=Treat bit field as an integer
  Extract Bits2 : simulink/Logic and Bit Operations/Extract Bits  SystemSampleTime=-1  bitsToExtract=Range of bits  numBits=8  bitIdxRange=[16 23]  outScalingMode=Treat bit field as an integer
  Extract Bits3 : simulink/Logic and Bit Operations/Extract Bits  SystemSampleTime=-1  bitsToExtract=Range of bits  numBits=8  bitIdxRange=[24 31]  outScalingMode=Treat bit field as an integer
  Extract Bits4 : simulink/Logic and Bit Operations/Extract Bits  SystemSampleTime=-1  bitsToExtract=Range of bits  numBits=8  bitIdxRange=[0 7]  outScalingMode=Treat bit field as an integer
  Extract Bits5 : simulink/Logic and Bit Operations/Extract Bits  SystemSampleTime=-1  bitsToExtract=Range of bits  numBits=8  bitIdxRange=[8 15]  outScalingMode=Treat bit field as an integer
  Extract Bits6 : simulink/Logic and Bit Operations/Extract Bits  SystemSampleTime=-1  bitsToExtract=Range of bits  numBits=8  bitIdxRange=[16 23]  outScalingMode=Treat bit field as an integer
  Extract Bits7 : simulink/Logic and Bit Operations/Extract Bits  SystemSampleTime=-1  bitsToExtract=Range of bits  numBits=8  bitIdxRange=[24 31]  outScalingMode=Treat bit field as an integer
  Mux : Mux  Inputs=8
  uint8 array : Outport
  wires:
  low-order uint32/1 -> Extract Bits/1, Extract Bits1/1, Extract Bits2/1, Extract Bits3/1
  Mux/1 -> uint8 array/1
  high-order uint1/1 -> Extract Bits4/1, Extract Bits5/1, Extract Bits6/1, Extract Bits7/1
  Extract Bits/1 -> Mux/1
  Extract Bits7/1 -> Mux/8
  Extract Bits1/1 -> Mux/2
  Extract Bits2/1 -> Mux/3
  Extract Bits3/1 -> Mux/4
  Extract Bits4/1 -> Mux/5
  Extract Bits5/1 -> Mux/6
  Extract Bits6/1 -> Mux/7

== system Main/Send ECAN1 Message/C-function Call ==
  parameters : Inport
  Enable : EnablePort
  ECAN1 Transmit : dsPICdrivers/OTHERS/C Function Call  Tag=dsPIC_dsPIC_CFunctionCall  fctName='ecan1_transmit_matlab'  INPUT_SIZE=8  INPUT1=uint16  INPUT2=--  INPUT3=--  OUTPUT_SIZE=1  OUTPUT1=--  SampleTime=c_func_sample_time  InputType=[ 4 ]  OutputType=[ ]  FctDeclaration=extern void ecan1_transmit_matlab(uint16_T* u1);  FctCall=ecan1_transmit_matlab(*%u1);  OrderingInOutPopup=None
  wires:
  parameters/1 -> ECAN1 Transmit/1

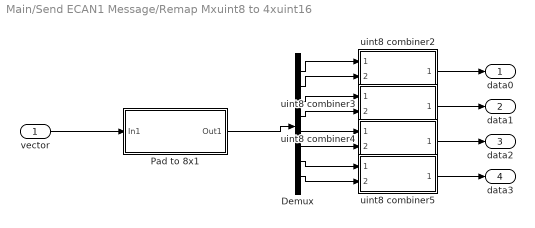
== system Main/Send ECAN1 Message/Remap Mxuint8 to 4xuint16 ==
  vector : Inport
  Demux : Demux  Outputs=8
  Pad to 8x1 : Subsystem
  uint8 combiner2 : Subsystem
  uint8 combiner3 : Subsystem
  uint8 combiner4 : Subsystem
  uint8 combiner5 : Subsystem
  data0 : Outport
  data1 : Outport  Port=2
  data2 : Outport  Port=3
  data3 : Outport  Port=4
  wires:
  Demux/8 -> uint8 combiner5/2(low-order)
  Demux/7 -> uint8 combiner5/1(high-order)
  Demux/6 -> uint8 combiner4/2(low-order)
  Demux/5 -> uint8 combiner4/1(high-order)
  Demux/4 -> uint8 combiner3/2(low-order)
  Demux/3 -> uint8 combiner3/1(high-order)
  Demux/2 -> uint8 combiner2/2(low-order)
  Demux/1 -> uint8 combiner2/1(high-order)
  Pad to 8x1/1(Out1) -> Demux/1
  uint8 combiner2/1(combined) -> data0/1
  uint8 combiner3/1(combined) -> data1/1
  vector/1 -> Pad to 8x1/1(In1)
  uint8 combiner4/1(combined) -> data2/1
  uint8 combiner5/1(combined) -> data3/1

== system Main/Send ECAN1 Message/uint8 combiner ==
  high-order : Inport
  low-order : Inport  Port=2
  Bitwise Operator : simulink/Logic and Bit Operations/Bitwise Operator  logicop=OR  UseBitMask=off  NumInputPorts=2  BitMask=bin2dec('11011001')  BitMaskRealWorld=Stored Integer
  Shift Arithmetic : simulink/Logic and Bit Operations/Shift Arithmetic  SystemSampleTime=-1  nBitShiftRight=-8  nBinPtShiftRight=0
  combined : Outport
  wires:
  Shift Arithmetic/1 -> Bitwise Operator/2
  high-order/1 -> Bitwise Operator/1
  Bitwise Operator/1 -> combined/1
  low-order/1 -> Shift Arithmetic/1

== system Main/Send ECAN1 Message/uint8 combiner1 ==
  high-order : Inport
  low-order : Inport  Port=2
  Bitwise Operator : simulink/Logic and Bit Operations/Bitwise Operator  logicop=OR  UseBitMask=off  NumInputPorts=2  BitMask=bin2dec('11011001')  BitMaskRealWorld=Stored Integer
  Shift Arithmetic : simulink/Logic and Bit Operations/Shift Arithmetic  SystemSampleTime=-1  nBitShiftRight=-8  nBinPtShiftRight=0
  combined : Outport
  wires:
  low-order/1 -> Shift Arithmetic/1
  Bitwise Operator/1 -> combined/1
  high-order/1 -> Bitwise Operator/1
  Shift Arithmetic/1 -> Bitwise Operator/2

== system Main/Send ECAN1 Message/Remap Mxuint8 to 4xuint16/Pad to 8x1 ==
  In1 : Inport
  Constant : Constant  Value=[0 0 0 0 0 0 0 0]  OutDataTypeMode=uint8
  Data Type Conversion : DataTypeConversion  OutDataTypeMode=uint16
  Merge : Merge  InitialOutput=[0 0 0 0 0 0 0 0]  AllowUnequalInputPortWidths=on
  Out1 : Outport
  wires:
  In1/1 -> Merge/1
  Merge/1 -> Data Type Conversion/1
  Constant/1 -> Merge/2
  Data Type Conversion/1 -> Out1/1

== system Main/Send ECAN1 Message/Remap Mxuint8 to 4xuint16/uint8 combiner2 ==
  high-order : Inport
  low-order : Inport  Port=2
  Bitwise Operator : simulink/Logic and Bit Operations/Bitwise Operator  logicop=OR  UseBitMask=off  NumInputPorts=2  BitMask=bin2dec('11011001')  BitMaskRealWorld=Stored Integer
  Shift Arithmetic : simulink/Logic and Bit Operations/Shift Arithmetic  SystemSampleTime=-1  nBitShiftRight=-8  nBinPtShiftRight=0
  combined : Outport
  wires:
  Shift Arithmetic/1 -> Bitwise Operator/2
  high-order/1 -> Bitwise Operator/1
  Bitwise Operator/1 -> combined/1
  low-order/1 -> Shift Arithmetic/1

== system Main/Send ECAN1 Message/Remap Mxuint8 to 4xuint16/uint8 combiner3 ==
  high-order : Inport
  low-order : Inport  Port=2
  Bitwise Operator : simulink/Logic and Bit Operations/Bitwise Operator  logicop=OR  UseBitMask=off  NumInputPorts=2  BitMask=bin2dec('11011001')  BitMaskRealWorld=Stored Integer
  Shift Arithmetic : simulink/Logic and Bit Operations/Shift Arithmetic  SystemSampleTime=-1  nBitShiftRight=-8  nBinPtShiftRight=0
  combined : Outport
  wires:
  low-order/1 -> Shift Arithmetic/1
  Bitwise Operator/1 -> combined/1
  high-order/1 -> Bitwise Operator/1
  Shift Arithmetic/1 -> Bitwise Operator/2

== system Main/Send ECAN1 Message/Remap Mxuint8 to 4xuint16/uint8 combiner4 ==
  high-order : Inport
  low-order : Inport  Port=2
  Bitwise Operator : simulink/Logic and Bit Operations/Bitwise Operator  logicop=OR  UseBitMask=off  NumInputPorts=2  BitMask=bin2dec('11011001')  BitMaskRealWorld=Stored Integer
  Shift Arithmetic : simulink/Logic and Bit Operations/Shift Arithmetic  SystemSampleTime=-1  nBitShiftRight=-8  nBinPtShiftRight=0
  combined : Outport
  wires:
  Shift Arithmetic/1 -> Bitwise Operator/2
  high-order/1 -> Bitwise Operator/1
  Bitwise Operator/1 -> combined/1
  low-order/1 -> Shift Arithmetic/1

== system Main/Send ECAN1 Message/Remap Mxuint8 to 4xuint16/uint8 combiner5 ==
  high-order : Inport
  low-order : Inport  Port=2
  Bitwise Operator : simulink/Logic and Bit Operations/Bitwise Operator  logicop=OR  UseBitMask=off  NumInputPorts=2  BitMask=bin2dec('11011001')  BitMaskRealWorld=Stored Integer
  Shift Arithmetic : simulink/Logic and Bit Operations/Shift Arithmetic  SystemSampleTime=-1  nBitShiftRight=-8  nBinPtShiftRight=0
  combined : Outport
  wires:
  low-order/1 -> Shift Arithmetic/1
  Bitwise Operator/1 -> combined/1
  high-order/1 -> Bitwise Operator/1
  Shift Arithmetic/1 -> Bitwise Operator/2

== matlab function Configure ECAN 1/Subsystem2/Embedded MATLAB Function ==
  settings: sampleTime=Inf
  data: u input inherited; y output inherited
function y = bitsetVector(u)

y = uint16(0);
for k = 1:size(u,1)
    y = bitset(y,u(k)+1);
end;

== matlab function Configure ECAN 1/Subsystem3/Embedded MATLAB Function ==
  settings: updateMethod=DISCRETE  sampleTime=Inf
  data: CiTR01CON output inherited; CiTR23CON output inherited; CiTR45CON output inherited; CiTR67CON output inherited; bufs input inherited; buf_priorities input inherited; buf_rtes input inherited
function [CiTR01CON, CiTR23CON, CiTR45CON, CiTR67CON] = buildCiTRmnCONReg(bufs, buf_priorities, buf_rtes)

% Create a vector of shorts to modify
regs = uint16(zeros(8,1));

% Go through all enabled transmission buffers setting appropriate bits
for b = 1:size(bufs,1)
    
    index = bufs(b);
    
    % Set transmission bit
    regs(index) = bitset(regs(index),8);
    
    % Set priority bits
    regs(index) = bitor(regs(index), uint16(buf_priorities(index)-1));
    
    % Set remote transmit enable bits
    if all(buf_rtes(index))
        regs(index) = bitset(regs(index),3);
    end
end

% Map our matrix into registers
CiTR01CON = uint16(bitshift(regs(2),8) | regs(1));
CiTR23CON = uint16(bitshift(regs(4),8) | regs(3));
CiTR45CON = uint16(bitshift(regs(6),8) | regs(5));
CiTR67CON = uint16(bitshift(regs(8),8) | regs(7));
